simulink model "QPSK"  (R2020a)
settings: Solver=VariableStepAuto  StartTime=0.0  StopTime=10.0  RelTol=1e-3
settings Model: Creator=AVS  LastModifiedBy=AVS

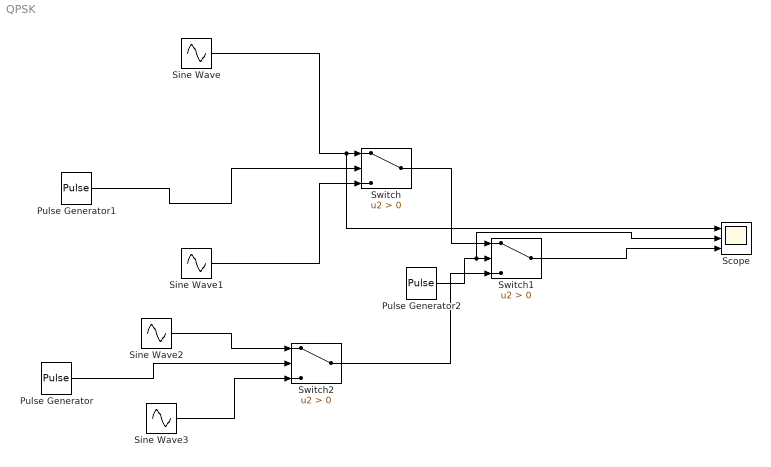
== system QPSK ==
  Pulse Generator : DiscretePulseGenerator  PulseType=Time based  PulseWidth=50
  Pulse Generator1 : DiscretePulseGenerator  PulseType=Time based  PulseWidth=50
  Pulse Generator2 : DiscretePulseGenerator  PulseType=Time based  Period=4  PulseWidth=50
  Scope : Scope  NumInputPorts=3
  Sine Wave : Sin  Frequency=2*pi*2  SampleTime=0.01
  Sine Wave1 : Sin  Frequency=2*pi*2  Phase=pi  SampleTime=0.01
  Sine Wave2 : Sin  Frequency=2*pi*2  Phase=pi/2  SampleTime=0.01
  Sine Wave3 : Sin  Frequency=2*pi*2  Phase=3*pi/2  SampleTime=0.01
  Switch : Switch  Criteria=u2 > Threshold
  Switch1 : Switch  Criteria=u2 > Threshold
  Switch2 : Switch  Criteria=u2 > Threshold
  wires:
  Pulse Generator1/1 -> Switch/2
  Sine Wave/1 -> Scope/1, Switch/1
  Sine Wave1/1 -> Switch/3
  Sine Wave2/1 -> Switch2/1
  Sine Wave3/1 -> Switch2/3
  Pulse Generator/1 -> Switch2/2
  Pulse Generator2/1 -> Scope/2, Switch1/2
  Switch/1 -> Switch1/1
  Switch2/1 -> Switch1/3
  Switch1/1 -> Scope/3
